simulink model "FEEDER_3_SC_TESTS"  (Simulink 8.1)
settings: Solver=ode1  StartTime=0.0  StopTime=15  FixedStep=Ts  MaxStep=1e-3  RelTol=1e-3
model workspace (MAT data in the model file):
  op_snapshot1 : opcond.OperatingPoint (value not decoded)
PostLoadFcn:
  | Ts=100e-6; BANSHEE_init;
InitFcn:
  | Ts=100e-6; BANSHEE_init;
undefined symbols (not defined in the file or in its folder): cable_spec, F3, Feeder3_lib, Left, relay_housing_lib, SM_UtilityService, SS_F3_RELAY_HOUSING, SS_Feeder3, type, utility_service_lib, V
libraries: breaker_lib x15, cables_lib x11, relay_modbus_lib x10, rtio_generic_modbus x10, artemis x8, transformer_lib x7, rtlab x6, Load_lib x5, ssn_lib x4, powerlib_extras x2, powerlib x2, LoadProfiles_lib x1
settings Model: ARTEMISmethode_block_infos=$$__separator__$$FEEDER_3_SC_TESTS/ARTEMIS Guide$$__separator__$$  Creator=RE25624  LastModifiedBy=RE25624  BufferReuse=off
settings SolverCC: ZeroCrossAlgorithm=Adaptive
settings DataIOCC: ExternalInput=getinputstruct(op_snapshot1)  InitialState=getstatestruct(op_snapshot1)  LimitDataPoints=off  MaxDataPoints=90060  SignalLoggingSaveFormat=Dataset  SaveOutput=off  SignalLogging=off  DSMLogging=off  SaveTime=off  OutputSaveName=result
settings OptimizationCC: BlockReduction=off  OptimizeBlockIOStorage=off  BufferReuse=off  ExpressionFolding=off  LocalBlockOutputs=off
settings DebuggingCC: MaxConsecutiveZCsMsg=warning  IgnoredZcDiagnostic=none  SolverPrmCheckMsg=none  MultiTaskRateTransMsg=warning  FcnCallInpInsideContextMsg=EnableAllAsWarning  FrameProcessingCompatibilityMsg=error  ModelReferenceExtraNoncontSigs=warning  StrictBusMsg=None
settings ModelReferenceCC: UpdateModelReferenceTargets=IfOutOfDate
settings SFSimCC: SFSimEcho=off
settings GRTTargetCC: CodeReplacementLibrary=C89/C90 (ANSI)

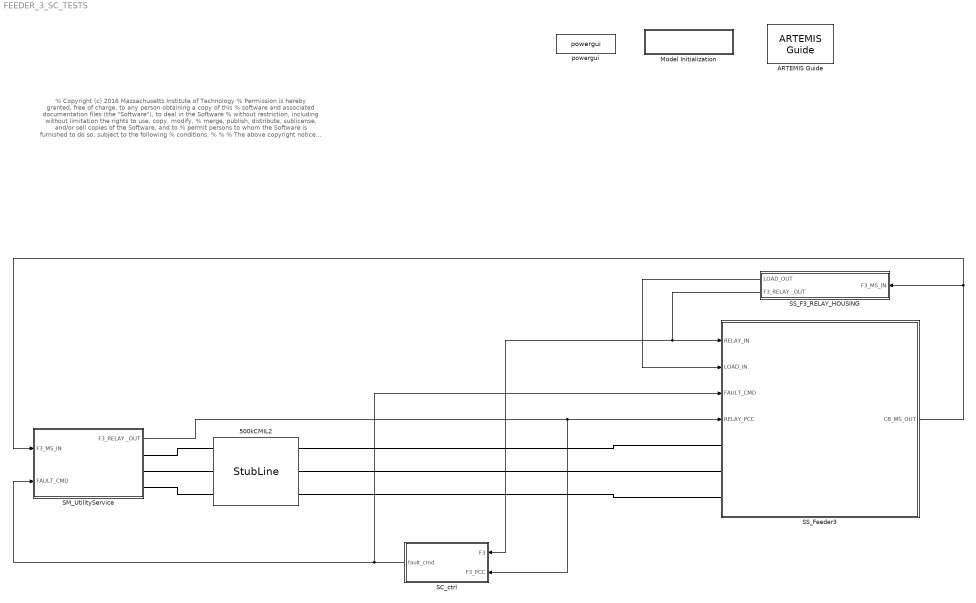
== system FEEDER_3_SC_TESTS ==
  note: % Copyright (c) 2016 Massachusetts Institute of Technology
      | % Permission is hereby granted, free of charge, to any person obtaining a copy of this
      | % software and associated documentation files (the "Software"), to deal in the Software
      | % without restriction, including without limitation the rights to use, copy, modify,
      | % merge, publish, distribute, sublicense, and/or sell copies of the Software, and to
      | % permit persons to whom the Software is furnished to do so, subject to the following
      | % conditions:
      | %
      | %
      | % The above copyright notice and this permission notice shall be included in
      | % all copies or substantial portions of the Software.
      | %
      | % THE SOFTWARE IS PROVIDED "AS IS", WITHOUT WARRANTY OF ANY KIND, EXPRESS OR IMPLIED,
      | % INCLUDING BUT NOT LIMITED TO THE WARRANTIES OF MERCHANTABILITY, FITNESS FOR A
      | % PARTICULAR PURPOSE AND NONINFRINGEMENT. IN NO EVENT SHALL THE AUTHORS OR COPYRIGHT
      | % HOLDERS BE LIABLE FOR ANY CLAIM, DAMAGES OR OTHER LIABILITY, WHETHER IN AN ACTION
      | % OF CONTRACT, TORT OR OTHERWISE, ARISING FROM, OUT OF OR IN CONNECTION WITH THE
      | % SOFTWARE OR THE USE OR OTHER DEALINGS IN THE SOFTWARE.
      | %
      | %
      | %%
  500kCMIL2 : artemis/ARTEMIS/StubLine  Phases=3  pu=off  L=10000 * 9.43453e-08 / 1  Lpu=0.08  R=10000 * 2.28409e-5 / 1  Rpu=0.002  S_base=450e6/3  V_base=230e3/sqrt(3)  F_base=60  Ts=Ts
  ARTEMIS Guide : artemis/ARTEMIS/ARTEMIS Guide  Tag=FTSSmethode_opal_4hx0r99  Description=5.0_z1  lock=on  Ts=Ts  opt=art5  dyna=off  nb_perm=4  RT_fullcomp=off  ssn=on  ssn_itvc=off  ssn_ivic=off  ssn_ext=off  ssn_solver=Art5 with Backward Euler nodal interface  ssn_impulse=off  ssn_quasimpulse=off  ssn_impulse_loop=5  paraExtinctionThy=off  Thy_Impulse=on  dtc=Off  dtc_opt=normal  ao=on  simtype=off  ct_mac=off  lin_mov=off  lsp=[0.001 2]  spike_skip=Disabled  dtc_extra=1  dtc_sws=normal  dtc_pied=0.5  SPSRulesBlock=SPSRules  tre=on  ctmm=off  LF=off  dpl_type=ARTEMiS DPL  rlc_type=off  custom_type=off  para=on  ssn_ImpulseLoopBlockedStateUpdate=5  ssn_mov_iter_number=5  ssn_switch_iter_number=5
  Model Initialization : Subsystem  AncestorBlock=artemis/Tools /Misc/Model Initialization  mask(Model Functions){InitFcnX=Ts=100e-6; BANSHEE_init;, prel=off, posl=on, inif=on, strf=off}
      mask prompts: InitFcnX "Initialisation"; prel "Preload Function"; posl "PostLoad Function"; inif "InitFcn"; strf "StartFcn"
      mask init:
      | currentBlock = gcb;
      | root = bdroot(currentBlock);
      | 
      | if ~strcmp(get_param(root,'BlockDiagramType'),'library')
      |     if prel==1
      |         set_param(root, 'PreLoadFcn', InitFcnX);
      |     else
      |         set_param(root, 'PreLoadFcn', '');
      |     end
      |     if inif==1
      |         set_param(root, 'InitFcn', InitFcnX);
      |     else
      |         set_param(root, 'InitFcn', '');
      |     end
      |     if strf==1
      |         set_param(root, 'StartFcn', InitFcnX);
      |     else
      |         set_param(root, 'StartFcn', '');
      |     end
      |     if posl==1
      |         set_param(root, 'PostLoadFcn', InitFcnX);
      |     else
      |         set_param(root, 'PostLoadFcn', '');
      |     end
      | end
      | 
      | pos = get_param(currentBlock, 'Position');
      | width = pos(3) - pos(1); height = pos(4) - pos(2);
      | txt = [ upper(root) '\n' '- InitFcn. . . . . '  get_param(root, 'InitFcn') ];
      settings: CopyFcn=set_param(gcb,'LinkStatus','inactive')
      mask Display: text(5, height*0.5, txt, 'horizontalAlignment', 'left', 'verticalAlignment', 'middle') ;
  SC_ctrl : Subsystem
  SM_UtilityService : Subsystem  AncestorBlock=utility_service_lib/SM_UtilityService
  SS_F3_RELAY_HOUSING : Subsystem  AncestorBlock=relay_housing_lib/SS_F3_RELAY_HOUSING
  SS_Feeder3 : Subsystem  AncestorBlock=Feeder3_lib/SS_Feeder3
  powergui : powerlib/powergui  Priority=2  SimulationMode=Discrete  SolverType=Tustin  SampleTime=Ts  frequency=60  SPID=off  DisableSnubberDevices=off  DisableRonSwitches=off  DisableVfSwitches=off  SwTol=0  Interpol=off  DisplayEquations=off  frequencyindice=0  Pbase=100e6  ErrMax=1e-4  Iterations=50  UnitsV=kV  UnitsW=MW  FunctionMessages=off  echomessages=off  HookPort=off  EnableUseOfTLC=off  x0status=blocks  RestoreLinks=warning  ResistiveCurrentMeasurement=off  Frange=logspace(0,3,50)  Ylog=off  Xlog=off  ShowGrid=off  save=off  variable=ZData  structure=0  ZoomFFT=on  StartTime=0.0  cycles=2  DisplayStyle=off  fundamental=60  FreqAxis=off  MaxFrequency=1000  frequencyindicesteady=1  RmsSteady=1  display=off  Ts=0  methode=off
  wires:
  SS_Feeder3/1(CB_MS_OUT) -> SS_F3_RELAY_HOUSING/1(F3_MS_IN), SM_UtilityService/1(F3_MS_IN)
  SS_F3_RELAY_HOUSING/2(F3_RELAY _OUT) -> SS_Feeder3/1(RELAY_IN), SC_ctrl/1(F3)
  SS_F3_RELAY_HOUSING/1(LOAD_OUT) -> SS_Feeder3/2(LOAD_IN)
  SC_ctrl/1(fault_cmd) -> SM_UtilityService/2(FAULT_CMD), SS_Feeder3/3(FAULT_CMD)
  SM_UtilityService/1(F3_RELAY _OUT) -> SC_ctrl/2(F3_PCC), SS_Feeder3/4(RELAY_PCC)
  connections:
  500kCMIL2/RConn3 -- SS_Feeder3/LConn3
  500kCMIL2/RConn2 -- SS_Feeder3/LConn2
  500kCMIL2/RConn1 -- SS_Feeder3/LConn1
  500kCMIL2/LConn2 -- SM_UtilityService/RConn2
  500kCMIL2/LConn1 -- SM_UtilityService/RConn1
  500kCMIL2/LConn3 -- SM_UtilityService/RConn3

== system FEEDER_3_SC_TESTS/Model Initialization ==

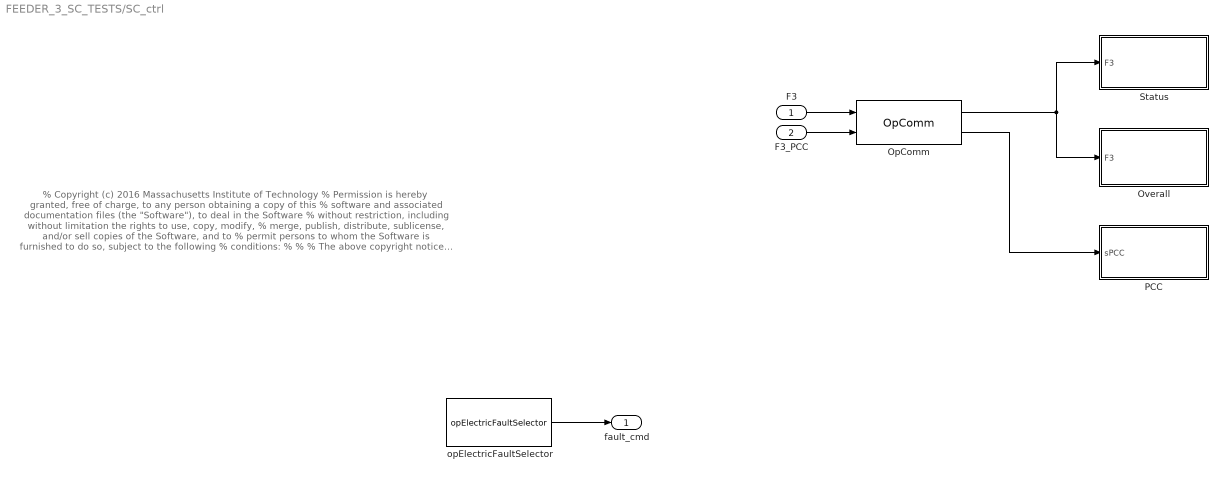
== system FEEDER_3_SC_TESTS/SC_ctrl ==
  note: % Copyright (c) 2016 Massachusetts Institute of Technology
      | % Permission is hereby granted, free of charge, to any person obtaining a copy of this
      | % software and associated documentation files (the "Software"), to deal in the Software
      | % without restriction, including without limitation the rights to use, copy, modify,
      | % merge, publish, distribute, sublicense, and/or sell copies of the Software, and to
      | % permit persons to whom the Software is furnished to do so, subject to the following
      | % conditions:
      | %
      | %
      | % The above copyright notice and this permission notice shall be included in
      | % all copies or substantial portions of the Software.
      | %
      | % THE SOFTWARE IS PROVIDED "AS IS", WITHOUT WARRANTY OF ANY KIND, EXPRESS OR IMPLIED,
      | % INCLUDING BUT NOT LIMITED TO THE WARRANTIES OF MERCHANTABILITY, FITNESS FOR A
      | % PARTICULAR PURPOSE AND NONINFRINGEMENT. IN NO EVENT SHALL THE AUTHORS OR COPYRIGHT
      | % HOLDERS BE LIABLE FOR ANY CLAIM, DAMAGES OR OTHER LIABILITY, WHETHER IN AN ACTION
      | % OF CONTRACT, TORT OR OTHERWISE, ARISING FROM, OUT OF OR IN CONNECTION WITH THE
      | % SOFTWARE OR THE USE OR OTHER DEALINGS IN THE SOFTWARE.
      | %
      | %
      | %%
  F3 : Inport
  F3_PCC : Inport  Port=2
  OpComm : rtlab/OpComm  nbport=2  groupe_acq=1  subsys_rate=0  st=0  Synchronization=on  Interpolation=on  Threshold=1.0  Missed_Data=off  Sim_Time=off  Samples=off  dynSigOut=off  from_console=0  warning_done=off  writeOpCommFile=off  Offset=off
  Overall : Subsystem
  PCC : Subsystem
  Status : Subsystem
  opElectricFaultSelector : artemis/Tools /POW faults/opElectricFaultSelector  phase_a=on  phase_b=on  phase_c=on  gnd_fault=on  Tacq=1  Tst=[0.1 0 10]  enable_POW=off  angle_POW=[15 0 10]  Tdr="[10.5 0  20]"  fault_location_menu=No fault  T_init=0.1
  fault_cmd : Outport
  wires:
  F3/1 -> OpComm/1
  OpComm/1 -> Overall/1(F3), Status/1(F3)
  opElectricFaultSelector/1 -> fault_cmd/1
  F3_PCC/1 -> OpComm/2
  OpComm/2 -> PCC/1(sPCC)

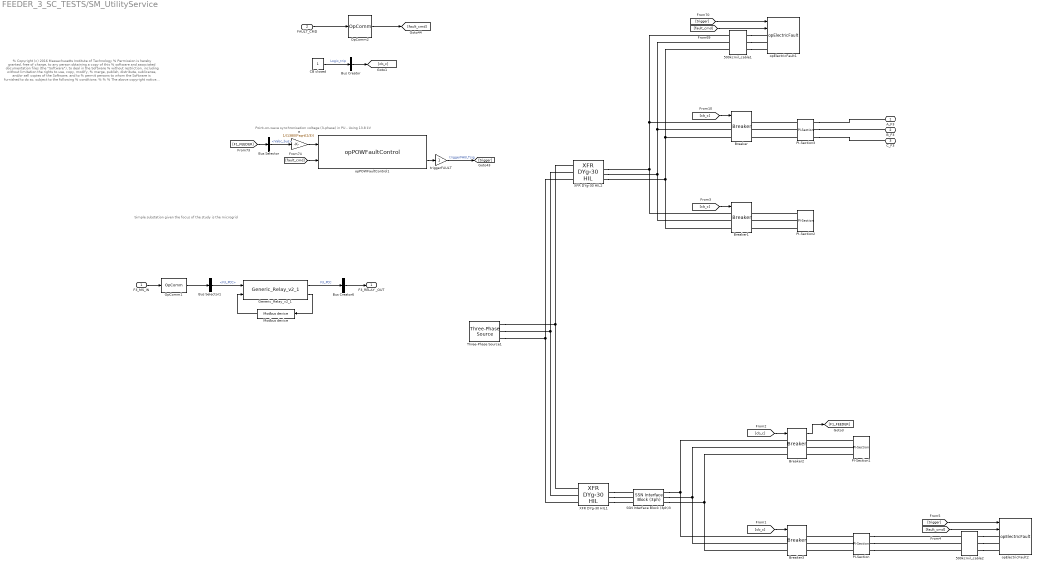
== system FEEDER_3_SC_TESTS/SM_UtilityService ==
  note: Simple substation given the focus of the study is the microgrid
  note: % Copyright (c) 2016 Massachusetts Institute of Technology
      | % Permission is hereby granted, free of charge, to any person obtaining a copy of this
      | % software and associated documentation files (the "Software"), to deal in the Software
      | % without restriction, including without limitation the rights to use, copy, modify,
      | % merge, publish, distribute, sublicense, and/or sell copies of the Software, and to
      | % permit persons to whom the Software is furnished to do so, subject to the following
      | % conditions:
      | %
      | %
      | % The above copyright notice and this permission notice shall be included in
      | % all copies or substantial portions of the Software.
      | %
      | % THE SOFTWARE IS PROVIDED "AS IS", WITHOUT WARRANTY OF ANY KIND, EXPRESS OR IMPLIED,
      | % INCLUDING BUT NOT LIMITED TO THE WARRANTIES OF MERCHANTABILITY, FITNESS FOR A
      | % PARTICULAR PURPOSE AND NONINFRINGEMENT. IN NO EVENT SHALL THE AUTHORS OR COPYRIGHT
      | % HOLDERS BE LIABLE FOR ANY CLAIM, DAMAGES OR OTHER LIABILITY, WHETHER IN AN ACTION
      | % OF CONTRACT, TORT OR OTHERWISE, ARISING FROM, OUT OF OR IN CONNECTION WITH THE
      | % SOFTWARE OR THE USE OR OTHER DEALINGS IN THE SOFTWARE.
      | %
      | %
      | %%
  note: Point-on-wave synchronisation voltage (3-phase) in PU - Using 13.8 kV
  F3_MS_IN : Inport
  FAULT_CMD : Inport  Port=2
  500kcmil_cable1 : cables_lib/500kcmil_cable  length=1  par_sets=1
  500kcmil_cable2 : cables_lib/500kcmil_cable  length=1  par_sets=1
  Breaker{,1..3} (4 alike) : breaker_lib/Breaker  Ts=Ts
  Bus Creator : BusCreator  Inputs=1
  Bus Creator6 : BusCreator  Inputs=1
  Bus Selector : BusSelector  OutputSignals=Vabc_bus
  Bus Selector1 : BusSelector  OutputSignals=F3_PCC
  CB closed : Constant
  Generic_Relay_v2_1 : relay_modbus_lib/Generic_Relay_v2_1  Ts=Ts  relay_settings=[F3(1,:)]
  Modbus device : rtio_generic_modbus/Modbus device  conf_name=F3_relay_cfg1.opal  conf_name_mask=F3_relay_cfg1.xls  sample_time=Ts
  OpComm1 : rtlab/OpComm  nbport=1  groupe_acq=1  subsys_rate=0  st=0  Synchronization=on  Interpolation=on  Threshold=1.0  Missed_Data=off  Sim_Time=off  Samples=off  dynSigOut=off  from_console=0  warning_done=off  writeOpCommFile=off  Offset=off
  OpComm2 : rtlab/OpComm  nbport=1  groupe_acq=1  subsys_rate=0  st=0  Synchronization=on  Interpolation=on  Threshold=1.0  Missed_Data=off  Sim_Time=off  Samples=off  dynSigOut=off  from_console=1  warning_done=off  writeOpCommFile=off  Offset=off
  PI-Section : cables_lib/PI-Section  cable_spec=[cable_spec(13, :)]  line_length=3000  parallel_sets=1
  PI-Section1 : cables_lib/PI-Section  cable_spec=[cable_spec(13, :)]  line_length=500  parallel_sets=1
  PI-Section2 : cables_lib/PI-Section  cable_spec=[cable_spec(13, :)]  line_length=500  parallel_sets=1
  PI-Section3 : cables_lib/PI-Section  cable_spec=[cable_spec(13, :)]  line_length=500  parallel_sets=1
  SSN Interface Block (3ph)3 : ssn_lib/SSN Interface Block (3ph)  nb_phase=3  nb_port=2  p1_type=V-type(Left)  p2_type=V-type (Right)  p3_type=V-type(Left)  p4_type=V-type(Left)  p5_type=V-type(Left)  p6_type=V-type(Left)  p7_type=V-type(Left)  p8_type=V-type(Left)  p9_type=V-type(Left)  p10_type=V-type(Left)  p11_type=V-type(Left)  p12_type=V-type(Left)  p13_type=V-type(Left)  p14_type=V-type(Left)  p15_type=V-type(Left)  p16_type=V-type(Left)  I_port_shunt_resistance=1e9
  Three-Phase Source1 : powerlib/Electrical Sources/Three-Phase Source  Voltage=115000  PhaseAngle=0  Frequency=60  InternalConnection=Yg  SpecifyImpedance=on  Resistance=0.8929  Inductance=16.58e-3  ShortCircuitLevel=100e6  BaseVoltage=115000  XRratio=30  BusType=swing  Pref=0  Qref=0  Qmin=-inf  Qmax=inf
  XFR DYg-30 HIL1 : transformer_lib/XFR DYg-30 HIL  Rating=50000  Vp=115000  Vs=13800  Z=15  XR=30
  XFR DYg-30 HIL2 : transformer_lib/XFR DYg-30 HIL  Rating=50000  Vp=115000  Vs=13800  Z=15  XR=30
  a : Gain  Gain=1/(13800*sqrt(2/3))
  opElectricFault1 : artemis/Tools /POW faults/opElectricFault  FaultLocation=location 7  FaultResistance=0.0001  GroundResistance=0.0001  InitialStates=[0 0 0]  SnubberResistance=1e6  SnubberCapacitance=inf
  opElectricFault2 : artemis/Tools /POW faults/opElectricFault  FaultLocation=location 8  FaultResistance=0.0001  GroundResistance=0.0001  InitialStates=[0 0 0]  SnubberResistance=1e6  SnubberCapacitance=inf
  opPOWFaultControl1 : artemis/Tools /POW faults/opPOWFaultControl  Ts=Ts  usePLL=off  Fgrid=60  PLL_k=[180 3200 1]  vol_sel=1: rising zero-corssing  SyncPhase_menu=A  T_acq=0.8
  triggerFAULT : Gain
  A_F3 : PMIOPort  Port=1  Side=Right
  B_F3 : PMIOPort  Port=2  Side=Right
  C_F3 : PMIOPort  Port=3  Side=Right
  F3_RELAY _OUT : Outport
  wires:
  [cb_c] -> Breaker2/1
  [cb_c] -> Breaker/1
  [cb_c] -> Breaker1/1
  [cb_c] -> Breaker3/1
  Bus Creator/1 -> [cb_c]
  CB closed/1 -> Bus Creator/1  "Logic_trip"
  [fault_cmd] -> opElectricFault1/2
  [trigger] -> opElectricFault1/1
  [fault_cmd] -> opPOWFaultControl1/2
  opPOWFaultControl1/2 -> triggerFAULT/1
  triggerFAULT/1 -> [trigger]  "triggerFAULTsig"
  [F1_FEEDER] -> Bus Selector/1
  Bus Selector/1 -> a/1  "<Vabc_bus>"
  a/1 -> opPOWFaultControl1/1
  OpComm2/1 -> [fault_cmd]
  FAULT_CMD/1 -> OpComm2/1
  Breaker2/1 -> [F1_FEEDER]
  [fault_cmd] -> opElectricFault2/2
  [trigger] -> opElectricFault2/1
  OpComm1/1 -> Bus Selector1/1
  Generic_Relay_v2_1/2 -> Modbus device/1
  Modbus device/1 -> Generic_Relay_v2_1/2
  F3_MS_IN/1 -> OpComm1/1
  Bus Selector1/1 -> Generic_Relay_v2_1/1  "<F3_PCC>"
  Generic_Relay_v2_1/1 -> Bus Creator6/1  "F3_PCC"
  Bus Creator6/1 -> F3_RELAY _OUT/1
  connections:
  PI-Section2/LConn1 -- Breaker1/RConn1
  PI-Section2/LConn3 -- Breaker1/RConn3
  PI-Section1/LConn1 -- Breaker2/RConn1
  PI-Section1/LConn2 -- Breaker2/RConn2
  PI-Section3/LConn1 -- Breaker/RConn1
  PI-Section1/LConn3 -- Breaker2/RConn3
  Breaker3/LConn2 -- SSN Interface Block (3ph)3/RConn2 -- Breaker2/LConn2
  PI-Section3/LConn2 -- Breaker/RConn2
  Breaker3/LConn3 -- SSN Interface Block (3ph)3/RConn3 -- Breaker2/LConn3
  PI-Section/LConn3 -- Breaker3/RConn3
  PI-Section2/LConn2 -- Breaker1/RConn2
  PI-Section/LConn1 -- Breaker3/RConn1
  Breaker3/LConn1 -- SSN Interface Block (3ph)3/RConn1 -- Breaker2/LConn1
  PI-Section3/LConn3 -- Breaker/RConn3
  Breaker1/LConn2 -- 500kcmil_cable1/LConn2 -- Breaker/LConn2 -- XFR DYg-30 HIL2/RConn2
  XFR DYg-30 HIL2/RConn1 -- Breaker1/LConn1 -- 500kcmil_cable1/LConn1 -- Breaker/LConn1
  Breaker1/LConn3 -- 500kcmil_cable1/LConn3 -- Breaker/LConn3 -- XFR DYg-30 HIL2/RConn3
  PI-Section/LConn2 -- Breaker3/RConn2
  PI-Section3/RConn3 -- C_F3/RConn1
  Three-Phase Source1/RConn3 -- XFR DYg-30 HIL2/LConn3 -- XFR DYg-30 HIL1/LConn3
  Three-Phase Source1/RConn2 -- XFR DYg-30 HIL2/LConn2 -- XFR DYg-30 HIL1/LConn2
  Three-Phase Source1/RConn1 -- XFR DYg-30 HIL2/LConn1 -- XFR DYg-30 HIL1/LConn1
  PI-Section3/RConn1 -- A_F3/RConn1
  PI-Section3/RConn2 -- B_F3/RConn1
  500kcmil_cable1/RConn3 -- opElectricFault1/LConn3
  500kcmil_cable1/RConn2 -- opElectricFault1/LConn2
  500kcmil_cable1/RConn1 -- opElectricFault1/LConn1
  500kcmil_cable2/RConn3 -- opElectricFault2/LConn3
  500kcmil_cable2/RConn2 -- opElectricFault2/LConn2
  500kcmil_cable2/RConn1 -- opElectricFault2/LConn1
  PI-Section/RConn3 -- 500kcmil_cable2/LConn3
  PI-Section/RConn2 -- 500kcmil_cable2/LConn2
  PI-Section/RConn1 -- 500kcmil_cable2/LConn1
  XFR DYg-30 HIL1/RConn3 -- SSN Interface Block (3ph)3/LConn3
  XFR DYg-30 HIL1/RConn2 -- SSN Interface Block (3ph)3/LConn2
  XFR DYg-30 HIL1/RConn1 -- SSN Interface Block (3ph)3/LConn1

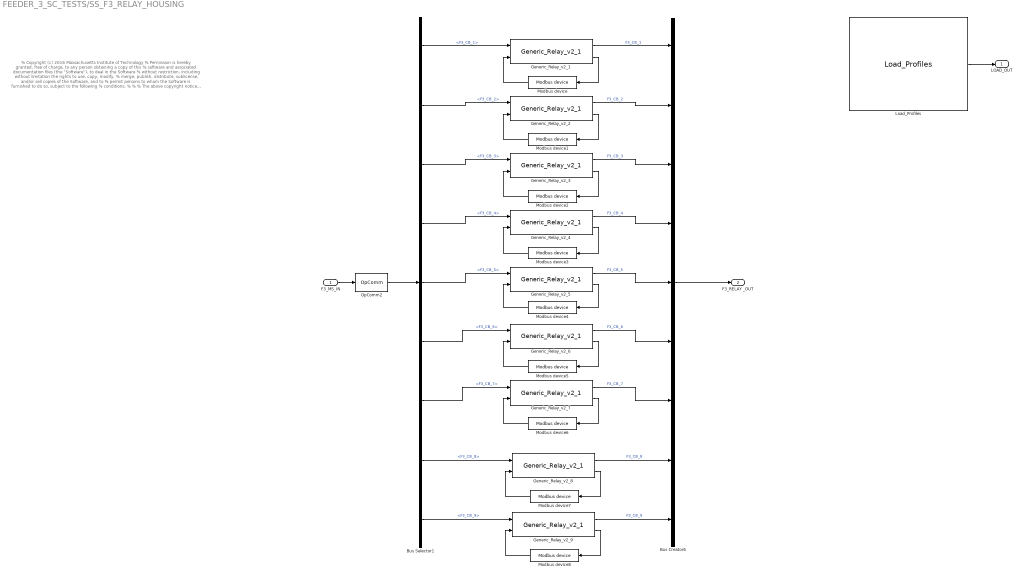
== system FEEDER_3_SC_TESTS/SS_F3_RELAY_HOUSING ==
  note: % Copyright (c) 2016 Massachusetts Institute of Technology
      | % Permission is hereby granted, free of charge, to any person obtaining a copy of this
      | % software and associated documentation files (the "Software"), to deal in the Software
      | % without restriction, including without limitation the rights to use, copy, modify,
      | % merge, publish, distribute, sublicense, and/or sell copies of the Software, and to
      | % permit persons to whom the Software is furnished to do so, subject to the following
      | % conditions:
      | %
      | %
      | % The above copyright notice and this permission notice shall be included in
      | % all copies or substantial portions of the Software.
      | %
      | % THE SOFTWARE IS PROVIDED "AS IS", WITHOUT WARRANTY OF ANY KIND, EXPRESS OR IMPLIED,
      | % INCLUDING BUT NOT LIMITED TO THE WARRANTIES OF MERCHANTABILITY, FITNESS FOR A
      | % PARTICULAR PURPOSE AND NONINFRINGEMENT. IN NO EVENT SHALL THE AUTHORS OR COPYRIGHT
      | % HOLDERS BE LIABLE FOR ANY CLAIM, DAMAGES OR OTHER LIABILITY, WHETHER IN AN ACTION
      | % OF CONTRACT, TORT OR OTHERWISE, ARISING FROM, OUT OF OR IN CONNECTION WITH THE
      | % SOFTWARE OR THE USE OR OTHER DEALINGS IN THE SOFTWARE.
      | %
      | %
      | %%
  F3_MS_IN : Inport
  Bus Creator6 : BusCreator  Inputs=9
  Bus Selector1 : BusSelector  OutputSignals=F3_CB_1,F3_CB_2,F3_CB_3,F3_CB_4,F3_CB_5,F3_CB_6,F3_CB_7,F3_CB_8,F3_CB_9
  Generic_Relay_v2_1 : relay_modbus_lib/Generic_Relay_v2_1  Ts=Ts  relay_settings=[F3(1,:)]
  Generic_Relay_v2_2 : relay_modbus_lib/Generic_Relay_v2_1  Ts=Ts  relay_settings=[F3(2,:)]
  Generic_Relay_v2_3 : relay_modbus_lib/Generic_Relay_v2_1  Ts=Ts  relay_settings=[F3(3,:)]
  Generic_Relay_v2_4 : relay_modbus_lib/Generic_Relay_v2_1  Ts=Ts  relay_settings=[F3(4,:)]
  Generic_Relay_v2_5 : relay_modbus_lib/Generic_Relay_v2_1  Ts=Ts  relay_settings=[F3(5,:)]
  Generic_Relay_v2_6 : relay_modbus_lib/Generic_Relay_v2_1  Ts=Ts  relay_settings=[F3(6,:)]
  Generic_Relay_v2_7 : relay_modbus_lib/Generic_Relay_v2_1  Ts=Ts  relay_settings=[F3(7,:)]
  Generic_Relay_v2_8 : relay_modbus_lib/Generic_Relay_v2_1  Ts=Ts  relay_settings=[F3(8,:)]
  Generic_Relay_v2_9 : relay_modbus_lib/Generic_Relay_v2_1  Ts=Ts  relay_settings=[F3(9,:)]
  Load_Profiles : LoadProfiles_lib/Load_Profiles
  Modbus device : rtio_generic_modbus/Modbus device  conf_name=F3_relay_cfg1.opal  conf_name_mask=F3_relay_cfg1.xls  sample_time=Ts
  Modbus device1 : rtio_generic_modbus/Modbus device  conf_name=F3_relay_cfg2.opal  conf_name_mask=F3_relay_cfg2.xls  sample_time=Ts
  Modbus device2 : rtio_generic_modbus/Modbus device  conf_name=F3_relay_cfg3.opal  conf_name_mask=F3_relay_cfg3.xls  sample_time=Ts
  Modbus device3 : rtio_generic_modbus/Modbus device  conf_name=F3_relay_cfg4.opal  conf_name_mask=F3_relay_cfg4.xls  sample_time=Ts
  Modbus device4 : rtio_generic_modbus/Modbus device  conf_name=F3_relay_cfg5.opal  conf_name_mask=F3_relay_cfg5.xls  sample_time=Ts
  Modbus device5 : rtio_generic_modbus/Modbus device  conf_name=F3_relay_cfg6.opal  conf_name_mask=F3_relay_cfg6.xls  sample_time=Ts
  Modbus device6 : rtio_generic_modbus/Modbus device  conf_name=F3_relay_cfg7.opal  conf_name_mask=F3_relay_cfg7.xls  sample_time=Ts
  Modbus device7 : rtio_generic_modbus/Modbus device  conf_name=F3_relay_cfg8.opal  conf_name_mask=F3_relay_cfg8.xls  sample_time=Ts
  Modbus device8 : rtio_generic_modbus/Modbus device  conf_name=F3_relay_cfg9.opal  conf_name_mask=F3_relay_cfg9.xls  sample_time=Ts
  OpComm2 : rtlab/OpComm  nbport=1  groupe_acq=1  subsys_rate=0  st=0  Synchronization=on  Interpolation=on  Threshold=1.0  Missed_Data=off  Sim_Time=off  Samples=off  dynSigOut=off  from_console=0  warning_done=off  writeOpCommFile=off  Offset=off
  LOAD_OUT : Outport
  F3_RELAY _OUT : Outport  Port=2
  wires:
  Load_Profiles/1 -> LOAD_OUT/1
  OpComm2/1 -> Bus Selector1/1
  Generic_Relay_v2_1/2 -> Modbus device/1
  Modbus device/1 -> Generic_Relay_v2_1/2
  Generic_Relay_v2_2/2 -> Modbus device1/1
  Modbus device1/1 -> Generic_Relay_v2_2/2
  Modbus device2/1 -> Generic_Relay_v2_3/2
  Generic_Relay_v2_3/2 -> Modbus device2/1
  Generic_Relay_v2_4/2 -> Modbus device3/1
  Modbus device3/1 -> Generic_Relay_v2_4/2
  Generic_Relay_v2_5/2 -> Modbus device4/1
  Modbus device4/1 -> Generic_Relay_v2_5/2
  Modbus device5/1 -> Generic_Relay_v2_6/2
  Generic_Relay_v2_6/2 -> Modbus device5/1
  Generic_Relay_v2_7/2 -> Modbus device6/1
  Modbus device6/1 -> Generic_Relay_v2_7/2
  F3_MS_IN/1 -> OpComm2/1
  Bus Selector1/1 -> Generic_Relay_v2_1/1  "<F3_CB_1>"
  Bus Selector1/2 -> Generic_Relay_v2_2/1  "<F3_CB_2>"
  Bus Selector1/3 -> Generic_Relay_v2_3/1  "<F3_CB_3>"
  Bus Selector1/4 -> Generic_Relay_v2_4/1  "<F3_CB_4>"
  Bus Selector1/5 -> Generic_Relay_v2_5/1  "<F3_CB_5>"
  Bus Selector1/6 -> Generic_Relay_v2_6/1  "<F3_CB_6>"
  Bus Selector1/7 -> Generic_Relay_v2_7/1  "<F3_CB_7>"
  Generic_Relay_v2_1/1 -> Bus Creator6/1  "F3_CB_1"
  Generic_Relay_v2_2/1 -> Bus Creator6/2  "F3_CB_2"
  Generic_Relay_v2_3/1 -> Bus Creator6/3  "F3_CB_3"
  Generic_Relay_v2_4/1 -> Bus Creator6/4  "F3_CB_4"
  Generic_Relay_v2_5/1 -> Bus Creator6/5  "F3_CB_5"
  Generic_Relay_v2_6/1 -> Bus Creator6/6  "F3_CB_6"
  Generic_Relay_v2_7/1 -> Bus Creator6/7  "F3_CB_7"
  Bus Creator6/1 -> F3_RELAY _OUT/1
  Modbus device7/1 -> Generic_Relay_v2_8/2
  Generic_Relay_v2_8/2 -> Modbus device7/1
  Generic_Relay_v2_9/2 -> Modbus device8/1
  Modbus device8/1 -> Generic_Relay_v2_9/2
  Generic_Relay_v2_8/1 -> Bus Creator6/8  "F3_CB_8"
  Generic_Relay_v2_9/1 -> Bus Creator6/9  "F3_CB_9"
  Bus Selector1/9 -> Generic_Relay_v2_9/1  "<F3_CB_9>"
  Bus Selector1/8 -> Generic_Relay_v2_8/1  "<F3_CB_8>"

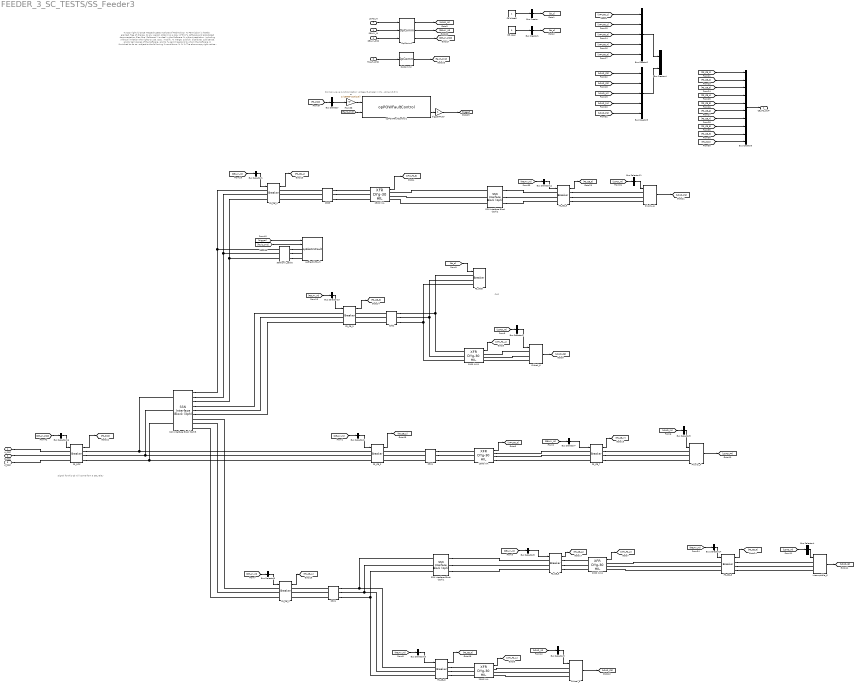
== system FEEDER_3_SC_TESTS/SS_Feeder3 ==
  note: Signal for this Cb will come from a SEL relay
  note: CHP
  note: % Copyright (c) 2016 Massachusetts Institute of Technology
      | % Permission is hereby granted, free of charge, to any person obtaining a copy of this
      | % software and associated documentation files (the "Software"), to deal in the Software
      | % without restriction, including without limitation the rights to use, copy, modify,
      | % merge, publish, distribute, sublicense, and/or sell copies of the Software, and to
      | % permit persons to whom the Software is furnished to do so, subject to the following
      | % conditions:
      | %
      | %
      | % The above copyright notice and this permission notice shall be included in
      | % all copies or substantial portions of the Software.
      | %
      | % THE SOFTWARE IS PROVIDED "AS IS", WITHOUT WARRANTY OF ANY KIND, EXPRESS OR IMPLIED,
      | % INCLUDING BUT NOT LIMITED TO THE WARRANTIES OF MERCHANTABILITY, FITNESS FOR A
      | % PARTICULAR PURPOSE AND NONINFRINGEMENT. IN NO EVENT SHALL THE AUTHORS OR COPYRIGHT
      | % HOLDERS BE LIABLE FOR ANY CLAIM, DAMAGES OR OTHER LIABILITY, WHETHER IN AN ACTION
      | % OF CONTRACT, TORT OR OTHERWISE, ARISING FROM, OUT OF OR IN CONNECTION WITH THE
      | % SOFTWARE OR THE USE OR OTHER DEALINGS IN THE SOFTWARE.
      | %
      | %
      | %%
  note: Point-on-wave synchronisation voltage (3-phase) in PU - Using 13.8 kV
  RELAY_IN : Inport
  LOAD_IN : Inport  Port=2
  FAULT_CMD : Inport  Port=3
  RELAY_PCC : Inport  Port=4
  1000 kVA : transformer_lib/XFR DYg-30 HIL  Rating=1000  Vp=13800  Vs=480  Z=5.56  XR=5.49
  1000 kVA1 : transformer_lib/XFR DYg-30 HIL  Rating=1000  Vp=13800  Vs=480  Z=5.56  XR=5.49
  2000 kVA : transformer_lib/XFR DYg-30 HIL  Rating=2000  Vp=13800  Vs=480  Z=5.75  XR=5.7
  2000 kVA1 : transformer_lib/XFR DYg-30 HIL  Rating=2000  Vp=13800  Vs=480  Z=5.75  XR=5.7
  2500 kVA : transformer_lib/XFR DYg-30 HIL  Rating=2500  Vp=13800  Vs=480  Z=5.75  XR=6.6
  500kcmil_cable : cables_lib/500kcmil_cable  length=1  par_sets=1
  Bus Creator : BusCreator  Inputs=1
  Bus Creator1 : BusCreator  Inputs=1
  Bus Creator2 : BusCreator  Inputs=5
  Bus Creator3 : BusCreator  Inputs=5
  Bus Creator4 : BusCreator  Inputs=2
  Bus Creator5 : BusCreator  Inputs=10
  Bus Selector : BusSelector  OutputSignals=Vabc_bus
  Bus Selector1 : BusSelector  OutputSignals=F3_CB_4
  Bus Selector10 : BusSelector  OutputSignals=F3_CB_5
  Bus Selector11 : BusSelector  OutputSignals=P6
  Bus Selector12 : BusSelector  OutputSignals=F3_CB_9
  Bus Selector13 : BusSelector  OutputSignals=F3_CB_3
  Bus Selector14 : BusSelector  OutputSignals=F3_CB_8
  Bus Selector16 : BusSelector  OutputSignals=F3_PCC
  Bus Selector2 : BusSelector  OutputSignals=C6
  Bus Selector3 : BusSelector  OutputSignals=P4
  Bus Selector4 : BusSelector  OutputSignals=I6
  Bus Selector5 : BusSelector  OutputSignals=C5
  Bus Selector6 : BusSelector  OutputSignals=F3_CB_2
  Bus Selector7 : BusSelector  OutputSignals=F3_CB_7
  Bus Selector8 : BusSelector  OutputSignals=F3_CB_6
  Bus Selector9 : BusSelector  OutputSignals=F3_CB_1
  C301 : cables_lib/PI-Section  cable_spec=[cable_spec(13, :)]  line_length=2500  parallel_sets=1
  C302 : cables_lib/PI-Section  cable_spec=[cable_spec(11, :)]  line_length=2000  parallel_sets=1
  C303 : cables_lib/PI-Section  cable_spec=[cable_spec(13, :)]  line_length=2000  parallel_sets=1
  C304 : cables_lib/PI-Section  cable_spec=[cable_spec(11, :)]  line_length=1500  parallel_sets=2
  CB closed : Constant
  CB open : Constant  Value=0
  Critical_5 : Load_lib/Dynamic_Load  V=460  Ts=Ts
  Critical_6 : Load_lib/Dynamic_Load  V=460  Ts=Ts
  F3_CB_{1..9} (9 alike) : breaker_lib/Breaker  Ts=Ts
  F3_GCB : breaker_lib/Breaker  Ts=Ts
  F3_PCC : breaker_lib/Breaker  Ts=Ts
  Interruptible_6 : Load_lib/Dynamic_Load  V=460  Ts=Ts
  OpComm1 : rtlab/OpComm  nbport=3  groupe_acq=1  subsys_rate=0  st=0  Synchronization=on  Interpolation=on  Threshold=1.0  Missed_Data=off  Sim_Time=off  Samples=off  dynSigOut=off  from_console=0  warning_done=off  writeOpCommFile=off  Offset=off
  OpComm2 : rtlab/OpComm  nbport=1  groupe_acq=1  subsys_rate=0  st=0  Synchronization=on  Interpolation=on  Threshold=1.0  Missed_Data=off  Sim_Time=off  Samples=off  dynSigOut=off  from_console=1  warning_done=off  writeOpCommFile=off  Offset=off
  Priority_4 : Load_lib/Dynamic_Load  V=460  Ts=Ts
  Priority_6 : Load_lib/Dynamic_Load  V=460  Ts=Ts
  SSN Interface Block (3ph)1 : ssn_lib/SSN Interface Block (3ph)  nb_phase=3  nb_port=2  p1_type=V-type(Left)  p2_type=V-type (Right)  p3_type=V-type(Left)  p4_type=V-type(Left)  p5_type=V-type(Left)  p6_type=V-type(Left)  p7_type=V-type(Left)  p8_type=V-type(Left)  p9_type=V-type(Left)  p10_type=V-type(Left)  p11_type=V-type(Left)  p12_type=V-type(Left)  p13_type=V-type(Left)  p14_type=V-type(Left)  p15_type=V-type(Left)  p16_type=V-type(Left)  I_port_shunt_resistance=1e9
  SSN Interface Block (3ph)2 : ssn_lib/SSN Interface Block (3ph)  nb_phase=3  nb_port=2  p1_type=V-type(Left)  p2_type=V-type (Right)  p3_type=V-type(Left)  p4_type=V-type(Left)  p5_type=V-type(Left)  p6_type=V-type(Left)  p7_type=V-type(Left)  p8_type=V-type(Left)  p9_type=V-type(Left)  p10_type=V-type(Left)  p11_type=V-type(Left)  p12_type=V-type(Left)  p13_type=V-type(Left)  p14_type=V-type(Left)  p15_type=V-type(Left)  p16_type=V-type(Left)  I_port_shunt_resistance=1e9
  SSN Interface Block (3ph)5 : ssn_lib/SSN Interface Block (3ph)  nb_phase=3  nb_port=4  p1_type=V-type(Left)  p2_type=V-type (Right)  p3_type=V-type (Right)  p4_type=V-type (Right)  p5_type=V-type(Left)  p6_type=V-type(Left)  p7_type=V-type(Left)  p8_type=V-type(Left)  p9_type=V-type(Left)  p10_type=V-type(Left)  p11_type=V-type(Left)  p12_type=V-type(Left)  p13_type=V-type(Left)  p14_type=V-type(Left)  p15_type=V-type(Left)  p16_type=V-type(Left)  I_port_shunt_resistance=1e9
  a : Gain  Gain=1/(13800*sqrt(2/3))
  opElectricFault : artemis/Tools /POW faults/opElectricFault  FaultLocation=location 4  FaultResistance=0.0001  GroundResistance=0.0001  InitialStates=[0 0 0]  SnubberResistance=1e6  SnubberCapacitance=inf
  opPOWFaultControl1 : artemis/Tools /POW faults/opPOWFaultControl  Ts=Ts  usePLL=off  Fgrid=60  PLL_k=[180 3200 1]  vol_sel=1: rising zero-corssing  SyncPhase_menu=A  T_acq=0.8
  triggerFAULT : Gain
  A_PCC : PMIOPort  Port=1  Side=Left
  B_PCC : PMIOPort  Port=2  Side=Left
  C_PCC : PMIOPort  Port=3  Side=Left
  CB_MS_OUT : Outport
  wires:
  CB closed/1 -> Bus Creator/1  "Logic_trip"
  Bus Creator/1 -> [cb_c]
  Bus Creator1/1 -> [cb_o]
  Bus Selector1/1 -> F3_CB_4/1  "<F3_CB_4>"
  CB open/1 -> Bus Creator1/1  "Logic_trip"
  LOAD_IN/1 -> OpComm1/1
  OpComm1/1 -> [LOAD_IN]
  [LOAD_IN] -> Bus Selector2/1
  [LOAD_IN] -> Bus Selector3/1
  [LOAD_IN] -> Bus Selector4/1
  [LOAD_IN] -> Bus Selector5/1
  Bus Selector2/1 -> Critical_6/1  "<C6>"
  Bus Selector3/1 -> Priority_4/1  "<P4>"
  Bus Selector4/1 -> Interruptible_6/1  "<I6>"
  Bus Selector5/1 -> Critical_5/1  "<C5>"
  2000 kVA/1 -> [XFM_F3_1]
  2000 kVA1/1 -> [XFM_F3_2]
  1000 kVA/1 -> [XFM_F3_3]
  1000 kVA1/1 -> [XFM_F3_4]
  [XFM_F3_2] -> Bus Creator2/2  "F3_X2"
  [XFM_F3_1] -> Bus Creator2/1  "F3_X1"
  [XFM_F3_5] -> Bus Creator2/5  "F3_X5"
  [XFM_F3_3] -> Bus Creator2/3  "F3_X3"
  [XFM_F3_4] -> Bus Creator2/4  "F3_X4"
  Critical_6/1 -> [LOAD_C6]
  Priority_4/1 -> [LOAD_P4]
  Interruptible_6/1 -> [LOAD_I6]
  Critical_5/1 -> [LOAD_C5]
  [LOAD_C6] -> Bus Creator3/2  "F3_C6"
  [LOAD_C5] -> Bus Creator3/1  "F3_C5"
  [LOAD_I6] -> Bus Creator3/3  "F3_I6"
  [LOAD_P4] -> Bus Creator3/4  "F3_P4"
  Bus Creator2/1 -> Bus Creator4/1  "XFR"
  Bus Creator3/1 -> Bus Creator4/2  "LOAD"
  F3_CB_4/1 -> [F3_CB_4]
  F3_CB_3/1 -> [F3_CB_3]
  F3_CB_2/1 -> [F3_CB_2]
  F3_CB_6/1 -> [F3_CB_6]
  F3_CB_1/1 -> [F3_CB_1]
  F3_CB_5/1 -> [F3_CB_5]
  [F3_CB_1] -> Bus Creator5/1  "F3_CB_1"
  [F3_CB_5] -> Bus Creator5/5  "F3_CB_5"
  [F3_CB_7] -> Bus Creator5/7  "F3_CB_7"
  [F3_CB_6] -> Bus Creator5/6  "F3_CB_6"
  [F3_CB_3] -> Bus Creator5/3  "F3_CB_3"
  [F3_CB_2] -> Bus Creator5/2  "F3_CB_2"
  [F3_CB_4] -> Bus Creator5/4  "F3_CB_4"
  Bus Creator5/1 -> CB_MS_OUT/1
  [RELAY_IN] -> Bus Selector1/1
  RELAY_IN/1 -> OpComm1/2
  OpComm1/2 -> [RELAY_IN]
  Bus Selector6/1 -> F3_CB_2/1  "<F3_CB_2>"
  [RELAY_IN] -> Bus Selector6/1
  Bus Selector7/1 -> F3_CB_7/1  "<F3_CB_7>"
  [RELAY_IN] -> Bus Selector7/1
  Bus Selector8/1 -> F3_CB_6/1  "<F3_CB_6>"
  [RELAY_IN] -> Bus Selector8/1
  Bus Selector9/1 -> F3_CB_1/1  "<F3_CB_1>"
  [RELAY_IN] -> Bus Selector9/1
  Bus Selector10/1 -> F3_CB_5/1  "<F3_CB_5>"
  [RELAY_IN] -> Bus Selector10/1
  Bus Selector13/1 -> F3_CB_3/1  "<F3_CB_3>"
  [RELAY_IN] -> Bus Selector13/1
  [cb_o] -> F3_GCB/1
  2500 kVA/1 -> [XFM_F3_5]
  F3_CB_7/1 -> [F3_CB_7]
  F3_PCC/1 -> [F3_PCC]
  [F3_PCC] -> Bus Creator5/10  "F3_PCC"
  [LOAD_IN] -> Bus Selector11/1
  Bus Selector11/1 -> Priority_6/1  "<P6>"
  Priority_6/1 -> [LOAD_P6]
  [LOAD_P6] -> Bus Creator3/5  "F3_P6"
  F3_CB_9/1 -> [F3_CB_9]
  Bus Selector12/1 -> F3_CB_9/1  "<F3_CB_9>"
  [RELAY_IN] -> Bus Selector12/1
  F3_CB_8/1 -> [F3_CB_8]
  Bus Selector14/1 -> F3_CB_8/1  "<F3_CB_8>"
  [RELAY_IN] -> Bus Selector14/1
  [F3_CB_8] -> Bus Creator5/8  "F3_CB_8"
  [F3_CB_9] -> Bus Creator5/9  "F3_CB_9"
  [fault_cmd] -> opPOWFaultControl1/2
  opPOWFaultControl1/2 -> triggerFAULT/1
  triggerFAULT/1 -> [trigger]  "triggerFAULTsig"
  [F3_PCC] -> Bus Selector/1
  Bus Selector/1 -> a/1  "<Vabc_bus>"
  a/1 -> opPOWFaultControl1/1
  [fault_cmd] -> opElectricFault/2
  [trigger] -> opElectricFault/1
  OpComm2/1 -> [fault_cmd]
  FAULT_CMD/1 -> OpComm2/1
  [RELAY_PCC] -> Bus Selector16/1
  OpComm1/3 -> [RELAY_PCC]
  RELAY_PCC/1 -> OpComm1/3
  Bus Selector16/1 -> F3_PCC/1  "<F3_PCC>"
  connections:
  F3_CB_5/LConn1 -- C301/RConn1 -- SSN Interface Block (3ph)1/LConn1
  F3_CB_6/RConn3 -- 2000 kVA1/LConn3
  Critical_6/LConn2 -- 1000 kVA1/RConn2
  C301/LConn2 -- F3_CB_1/RConn2
  Critical_6/LConn1 -- 1000 kVA1/RConn1
  F3_CB_5/LConn3 -- C301/RConn3 -- SSN Interface Block (3ph)1/LConn3
  Critical_6/LConn3 -- 1000 kVA1/RConn3
  C301/LConn3 -- F3_CB_1/RConn3
  C304/LConn1 -- F3_CB_2/RConn1
  1000 kVA1/LConn3 -- C302/RConn3 -- F3_GCB/LConn3
  C302/LConn2 -- F3_CB_3/RConn2
  1000 kVA1/LConn1 -- C302/RConn1 -- F3_GCB/LConn1
  F3_CB_6/RConn2 -- 2000 kVA1/LConn2
  1000 kVA1/LConn2 -- C302/RConn2 -- F3_GCB/LConn2
  C301/LConn1 -- F3_CB_1/RConn1
  F3_CB_5/RConn2 -- 2000 kVA/LConn2
  C302/LConn3 -- F3_CB_3/RConn3
  F3_CB_5/LConn2 -- C301/RConn2 -- SSN Interface Block (3ph)1/LConn2
  C304/LConn2 -- F3_CB_2/RConn2
  F3_CB_6/RConn1 -- 2000 kVA1/LConn1
  C302/LConn1 -- F3_CB_3/RConn1
  F3_CB_5/RConn1 -- 2000 kVA/LConn1
  F3_CB_5/RConn3 -- 2000 kVA/LConn3
  C304/LConn3 -- F3_CB_2/RConn3
  F3_CB_7/RConn1 -- Priority_4/LConn1
  F3_CB_7/RConn3 -- Priority_4/LConn3
  F3_CB_7/RConn2 -- Priority_4/LConn2
  F3_CB_8/LConn1 -- 2000 kVA1/RConn1
  F3_CB_8/LConn3 -- 2000 kVA1/RConn3
  F3_CB_8/LConn2 -- 2000 kVA1/RConn2
  Critical_5/LConn1 -- 2000 kVA/RConn1
  Critical_5/LConn3 -- 2000 kVA/RConn3
  Critical_5/LConn2 -- 2000 kVA/RConn2
  SSN Interface Block (3ph)2/LConn1 -- 2500 kVA/RConn1
  SSN Interface Block (3ph)2/LConn3 -- 2500 kVA/RConn3
  SSN Interface Block (3ph)2/LConn2 -- 2500 kVA/RConn2
  C304/RConn2 -- 1000 kVA/LConn2
  C304/RConn3 -- 1000 kVA/LConn3
  C304/RConn1 -- 1000 kVA/LConn1
  1000 kVA/RConn3 -- F3_CB_7/LConn3
  1000 kVA/RConn2 -- F3_CB_7/LConn2
  1000 kVA/RConn1 -- F3_CB_7/LConn1
  F3_CB_9/RConn1 -- Priority_6/LConn1
  F3_CB_9/RConn2 -- Priority_6/LConn2
  F3_CB_9/RConn3 -- Priority_6/LConn3
  F3_CB_8/RConn1 -- Interruptible_6/LConn1
  F3_CB_8/RConn2 -- Interruptible_6/LConn2
  F3_CB_8/RConn3 -- Interruptible_6/LConn3
  SSN Interface Block (3ph)5/RConn1 -- 500kcmil_cable/LConn1 -- F3_CB_4/LConn1
  SSN Interface Block (3ph)5/RConn3 -- 500kcmil_cable/LConn3 -- F3_CB_4/LConn3
  SSN Interface Block (3ph)5/RConn2 -- 500kcmil_cable/LConn2 -- F3_CB_4/LConn2
  SSN Interface Block (3ph)5/RConn4 -- F3_CB_3/LConn1
  SSN Interface Block (3ph)5/RConn6 -- F3_CB_3/LConn3
  SSN Interface Block (3ph)5/RConn5 -- F3_CB_3/LConn2
  F3_CB_1/LConn1 -- SSN Interface Block (3ph)5/RConn7
  F3_CB_1/LConn2 -- SSN Interface Block (3ph)5/RConn8
  F3_CB_1/LConn3 -- SSN Interface Block (3ph)5/RConn9
  SSN Interface Block (3ph)1/RConn2 -- F3_CB_6/LConn2
  SSN Interface Block (3ph)1/RConn1 -- F3_CB_6/LConn1
  SSN Interface Block (3ph)1/RConn3 -- F3_CB_6/LConn3
  C303/LConn1 -- F3_CB_4/RConn1
  C303/LConn2 -- F3_CB_4/RConn2
  C303/LConn3 -- F3_CB_4/RConn3
  C303/RConn2 -- 2500 kVA/LConn2
  C303/RConn3 -- 2500 kVA/LConn3
  C303/RConn1 -- 2500 kVA/LConn1
  F3_PCC/RConn1 -- F3_CB_2/LConn1 -- SSN Interface Block (3ph)5/LConn1
  F3_PCC/RConn3 -- F3_CB_2/LConn3 -- SSN Interface Block (3ph)5/LConn3
  F3_PCC/RConn2 -- F3_CB_2/LConn2 -- SSN Interface Block (3ph)5/LConn2
  500kcmil_cable/RConn2 -- opElectricFault/LConn2
  500kcmil_cable/RConn3 -- opElectricFault/LConn3
  500kcmil_cable/RConn1 -- opElectricFault/LConn1
  SSN Interface Block (3ph)2/RConn2 -- F3_CB_9/LConn2
  SSN Interface Block (3ph)2/RConn3 -- F3_CB_9/LConn3
  SSN Interface Block (3ph)2/RConn1 -- F3_CB_9/LConn1
  B_PCC/RConn1 -- F3_PCC/LConn2
  C_PCC/RConn1 -- F3_PCC/LConn3
  A_PCC/RConn1 -- F3_PCC/LConn1

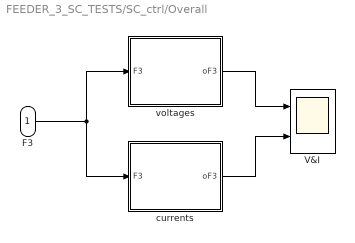
== system FEEDER_3_SC_TESTS/SC_ctrl/Overall ==
  F3 : Inport
  V&I : Scope  NumInputPorts=2
      settings: ShowLegends=on  TimeRange=10  YMin=0~0  YMax=1.4~80  SaveName=ScopeData3  Decimation=10
  currents : Subsystem
  voltages : Subsystem
  wires:
  F3/1 -> currents/1(F3), voltages/1(F3)
  voltages/1(oF3) -> V&I/1
  currents/1(oF3) -> V&I/2

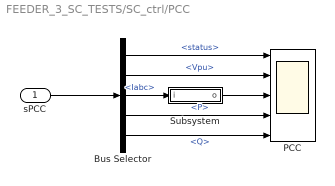
== system FEEDER_3_SC_TESTS/SC_ctrl/PCC ==
  sPCC : Inport
  Bus Selector : BusSelector  OutputSignals=F3_PCC.m.status,F3_PCC.m.Vpu,F3_PCC.m.Iabc,F3_PCC.m.P,F3_PCC.m.Q
  PCC : Scope  NumInputPorts=5
      settings: TimeRange=10  YMin=0~0~0~-250000~-2.5e+06  YMax=20~2.25~4500~2.25e+06~250000
  Subsystem : Subsystem
  wires:
  Bus Selector/3 -> Subsystem/1(i)  "<Iabc>"
  Bus Selector/5 -> PCC/5  "<Q>"
  Subsystem/1(o) -> PCC/3
  Bus Selector/4 -> PCC/4  "<P>"
  sPCC/1 -> Bus Selector/1
  Bus Selector/2 -> PCC/2  "<Vpu>"
  Bus Selector/1 -> PCC/1  "<status>"

== system FEEDER_3_SC_TESTS/SC_ctrl/Status ==
  F3 : Inport
  Bus Selector2 : BusSelector  OutputSignals=F3_CB_1.m.status,F3_CB_2.m.status,F3_CB_3.m.status,F3_CB_4.m.status,F3_CB_5.m.status,F3_CB_6.m.status,F3_CB_7.m.status,F3_CB_8.m.status,F3_CB_9.m.status
  Status : Scope  NumInputPorts=9
      settings: ShowLegends=on  TimeRange=0.4  YMin=7~7~7~7~7~7~7~7~7  YMax=7~7~7~7~7~7~7~7~7  SaveName=ScopeData3  Decimation=10
  wires:
  F3/1 -> Bus Selector2/1
  Bus Selector2/1 -> Status/1  "<status>"
  Bus Selector2/2 -> Status/2  "<status>"
  Bus Selector2/3 -> Status/3  "<status>"
  Bus Selector2/9 -> Status/9  "<status>"
  Bus Selector2/8 -> Status/8  "<status>"
  Bus Selector2/7 -> Status/7  "<status>"
  Bus Selector2/6 -> Status/6  "<status>"
  Bus Selector2/5 -> Status/5  "<status>"
  Bus Selector2/4 -> Status/4  "<status>"

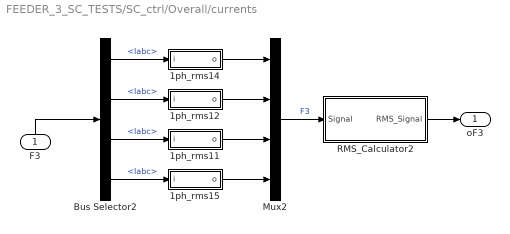
== system FEEDER_3_SC_TESTS/SC_ctrl/Overall/currents ==
  F3 : Inport
  1ph_rms11 : Subsystem
  1ph_rms12 : Subsystem
  1ph_rms14 : Subsystem
  1ph_rms15 : Subsystem
  Bus Selector2 : BusSelector  OutputSignals=F3_CB_1.m.Iabc,F3_CB_2.m.Iabc,F3_CB_3.m.Iabc,F3_CB_4.m.Iabc
  Mux2 : Mux
  RMS_Calculator2 : Subsystem
  oF3 : Outport
  wires:
  Mux2/1 -> RMS_Calculator2/1(Signal)  "F3"
  Bus Selector2/4 -> 1ph_rms15/1(i)  "<Iabc>"
  Bus Selector2/2 -> 1ph_rms12/1(i)  "<Iabc>"
  Bus Selector2/3 -> 1ph_rms11/1(i)  "<Iabc>"
  Bus Selector2/1 -> 1ph_rms14/1(i)  "<Iabc>"
  1ph_rms14/1(o) -> Mux2/1
  1ph_rms12/1(o) -> Mux2/2
  1ph_rms11/1(o) -> Mux2/3
  1ph_rms15/1(o) -> Mux2/4
  RMS_Calculator2/1(RMS_Signal) -> oF3/1
  F3/1 -> Bus Selector2/1

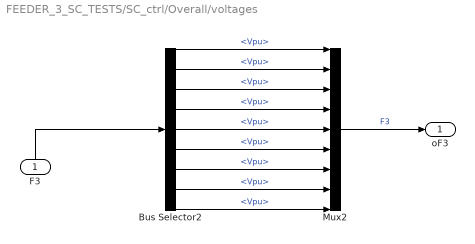
== system FEEDER_3_SC_TESTS/SC_ctrl/Overall/voltages ==
  F3 : Inport
  Bus Selector2 : BusSelector  OutputSignals=F3_CB_1.m.Vpu,F3_CB_2.m.Vpu,F3_CB_3.m.Vpu,F3_CB_4.m.Vpu,F3_CB_5.m.Vpu,F3_CB_6.m.Vpu,F3_CB_7.m.Vpu,F3_CB_8.m.Vpu,F3_CB_9.m.Vpu
  Mux2 : Mux  Inputs=9
  oF3 : Outport
  wires:
  Mux2/1 -> oF3/1  "F3"
  F3/1 -> Bus Selector2/1
  Bus Selector2/5 -> Mux2/5  "<Vpu>"
  Bus Selector2/4 -> Mux2/4  "<Vpu>"
  Bus Selector2/6 -> Mux2/6  "<Vpu>"
  Bus Selector2/3 -> Mux2/3  "<Vpu>"
  Bus Selector2/7 -> Mux2/7  "<Vpu>"
  Bus Selector2/8 -> Mux2/8  "<Vpu>"
  Bus Selector2/2 -> Mux2/2  "<Vpu>"
  Bus Selector2/9 -> Mux2/9  "<Vpu>"
  Bus Selector2/1 -> Mux2/1  "<Vpu>"

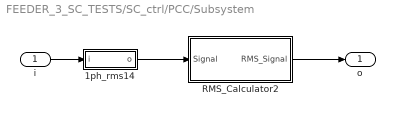
== system FEEDER_3_SC_TESTS/SC_ctrl/PCC/Subsystem ==
  i : Inport
  1ph_rms14 : Subsystem
  RMS_Calculator2 : Subsystem
  o : Outport
  wires:
  RMS_Calculator2/1(RMS_Signal) -> o/1
  i/1 -> 1ph_rms14/1(i)
  1ph_rms14/1(o) -> RMS_Calculator2/1(Signal)

== system FEEDER_3_SC_TESTS/SC_ctrl/Overall/currents/1ph_rms11 ==
  i : Inport
  Demux : Demux  Outputs=3
  o : Outport
  wires:
  Demux/1 -> o/1
  i/1 -> Demux/1

== system FEEDER_3_SC_TESTS/SC_ctrl/Overall/currents/1ph_rms12 ==
  i : Inport
  Demux : Demux  Outputs=3
  o : Outport
  wires:
  Demux/1 -> o/1
  i/1 -> Demux/1

== system FEEDER_3_SC_TESTS/SC_ctrl/Overall/currents/1ph_rms14 ==
  i : Inport
  Demux : Demux  Outputs=3
  o : Outport
  wires:
  Demux/1 -> o/1
  i/1 -> Demux/1

== system FEEDER_3_SC_TESTS/SC_ctrl/Overall/currents/1ph_rms15 ==
  i : Inport
  Demux : Demux  Outputs=3
  o : Outport
  wires:
  Demux/1 -> o/1
  i/1 -> Demux/1

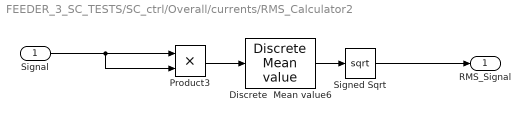
== system FEEDER_3_SC_TESTS/SC_ctrl/Overall/currents/RMS_Calculator2 ==
  Signal : Inport
  Discrete  Mean value6 : powerlib_extras/Discrete Measurements/Discrete  Mean value  Freq=60  Vinit=0  Ts=Ts
  Product3 : Product  RndMeth=Zero
  Signed Sqrt : Sqrt  SaturateOnIntegerOverflow=on
  RMS_Signal : Outport
  wires:
  Signed Sqrt/1 -> RMS_Signal/1
  Discrete  Mean value6/1 -> Signed Sqrt/1
  Product3/1 -> Discrete  Mean value6/1
  Signal/1 -> Product3/2, Product3/1

== system FEEDER_3_SC_TESTS/SC_ctrl/PCC/Subsystem/1ph_rms14 ==
  i : Inport
  Demux : Demux  Outputs=3
  o : Outport
  wires:
  Demux/1 -> o/1
  i/1 -> Demux/1

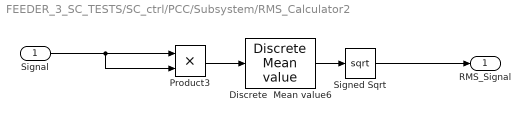
== system FEEDER_3_SC_TESTS/SC_ctrl/PCC/Subsystem/RMS_Calculator2 ==
  Signal : Inport
  Discrete  Mean value6 : powerlib_extras/Discrete Measurements/Discrete  Mean value  Freq=60  Vinit=0  Ts=Ts
  Product3 : Product  RndMeth=Zero
  Signed Sqrt : Sqrt  SaturateOnIntegerOverflow=on
  RMS_Signal : Outport
  wires:
  Signed Sqrt/1 -> RMS_Signal/1
  Discrete  Mean value6/1 -> Signed Sqrt/1
  Product3/1 -> Discrete  Mean value6/1
  Signal/1 -> Product3/2, Product3/1
